simulink model "ysw2_4"  (R2014a)
settings: Solver=ode45  StartTime=0.0  StopTime=10.0  RelTol=1e-3
settings Model: Creator=Administrator  LastModifiedBy=Administrator

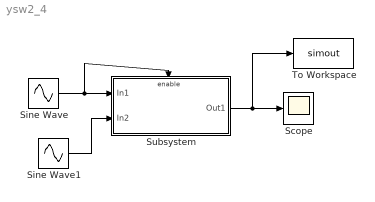
== system ysw2_4 ==
  Scope : Scope
  Sine Wave : Sin  SampleTime=0
  Sine Wave1 : Sin  SampleTime=0
  Subsystem : Subsystem
  To Workspace : ToWorkspace  VariableName=simout  SampleTime=-1
  wires:
  Sine Wave/1 -> Subsystem/Enable, Subsystem/1(In1)
  Sine Wave1/1 -> Subsystem/2(In2)
  Subsystem/1(Out1) -> To Workspace/1, Scope/1

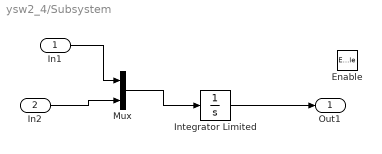
== system ysw2_4/Subsystem ==
  In1 : Inport
  In2 : Inport  Port=2
  Enable : EnablePort
  Integrator Limited : Integrator  LimitOutput=on  UpperSaturationLimit=1  LowerSaturationLimit=0
  Mux : Mux  Inputs=2
  Out1 : Outport
  wires:
  In1/1 -> Mux/1
  Mux/1 -> Integrator Limited/1
  Integrator Limited/1 -> Out1/1
  In2/1 -> Mux/2
